simulink model "realisticversion"  (R2020b)
settings: Solver=VariableStepAuto  StartTime=0.0  StopTime=0.1  MaxStep=1e-7  RelTol=1e-3
undefined symbols (not defined in the file): Acid, Lead
libraries: fl_lib x63, powerlib x24, nesl_utility x22, ee_lib x14, electricdrivelib x1, powerlib_meascontrol x1
settings Model: SimulationMode=accelerator  Creator=ahmet  LastModifiedBy=90554
settings SolverCC: ZeroCrossAlgorithm=Adaptive
settings DataIOCC: ReturnWorkspaceOutputs=off
settings DebuggingCC: IgnoredZcDiagnostic=none

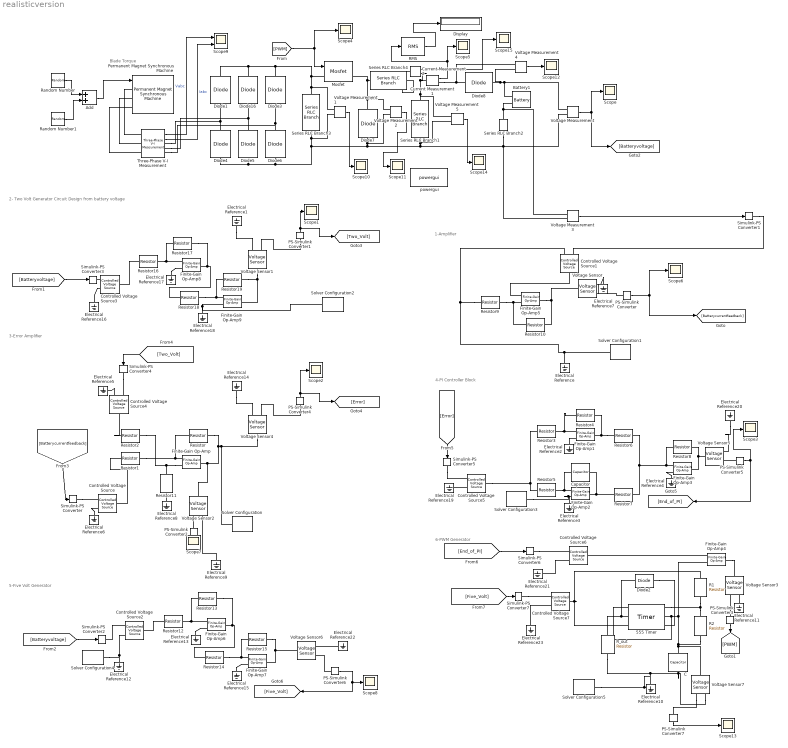
== system realisticversion ==
  note: 1-Amplifier
  note: 6-PWM Generator
  note: 5-Five Volt Generator
  note: 4-PI Controller Block
  note: 3-Error Amplifier
  note: 2- Two Volt Generator Circuit Design from battery voltage
  note: Blade Torque
  555 Timer : ee_lib/Integrated Circuits/Timer  V_CC=5 V  V_OL=0 V  V_OH=4.7 V  R_OUT=8 Ohm  Delay=1e-7 s  R_DIV=5 kOhm  R_closed=12 Ohm  R_open=5e+8 Ohm
      settings: SourceProductBaseCode=PS  InternalSimscapePortConfiguration="{\"Bottom\":[],\"Left\":[{\"id\":\"TRIG\",\"label\":\"TRIG\",\"type\":\"foundation.electrical.electrical\"},{\"id\":\"OUT\",\"label\":\"OUT\",\"type\":\"foundation.electrical.electrical\"},{\"id\":\"RESET\",\"label\":\"RESET\",\"type\":\"foundation.electrical.electrical\"}],\"Right\":[{\"id\":\"DISCH\",\"label\":\"DISCH\",\"type\":\"foundation.electrical.electrical\"},{\"id\":\"THRES\",\"label\":\"THRES\",\"type\":\"foundation.electrical.electrical\"},{\"id\":\"CONT\",\"label\":\"CONT\",\"type\":\"foundation.electrical.electrical\"}],\"Top\":[]}"
  Add : Sum
  Battery1 : electricdrivelib/Extra Sources/Battery  BatType=Lead-Acid  ShowTempParam=off  ThermalPreset=no  ShowAgeParam=off  NomV=24  NomQ=5.4  SOC=50  Batt_Tr=30  PresetModel=on  MaxQ=5.625  MinV=18  FullV=26.1316  Dis_rate=1.08  R=0.044444  Normal_OP=1.6755  expZone="[24.4342        0.018]"  current=[6.5 13 32.5]  Units=Time  Tci=20  NomT=20  T2=-30  MaxQ2=4.8  FullV2=7.1  Normal_OP2=5.655  expZone2="[6.58           1]"  Rca=0.6  ti=2000  Dp=0  Neq0=0  Tsim=1e6  Ta1=25  Qeol=5.4*0.9  Reol=0.013333*1.2  Char_age=[2.3478, 3]  Dis_age=[2.3478, 10]  N1=1500  N2=10500  N3=1000  N4=1400  Ta2=45  N5=950
  C : fl_lib/Electrical/Electrical Elements/Capacitor  c=1e-9 F  r=1e-6 Ohm  g=0 1/Ohm  i_specify=off  i_priority=None  i=0 A  i_nominal_specify=off  i_nominal_unit=A  i_nominal_value=1  v_specify=off  v_priority=None  v=0 V  v_nominal_specify=off  v_nominal_unit=V  v_nominal_value=1  vc_specify=off  vc_priority=High  vc=0 V  vc_nominal_specify=off  vc_nominal_unit=V  vc_nominal_value=1
  Capacitor : fl_lib/Electrical/Electrical Elements/Capacitor  c=3.3e-6 F  r=1e-6 Ohm  g=0 1/Ohm  i_specify=off  i_priority=None  i=0 A  i_nominal_specify=off  i_nominal_unit=A  i_nominal_value=1  v_specify=off  v_priority=None  v=0 V  v_nominal_specify=off  v_nominal_unit=V  v_nominal_value=1  vc_specify=off  vc_priority=High  vc=0 V  vc_nominal_specify=off  vc_nominal_unit=V  vc_nominal_value=1
  Controlled Voltage Source{,1..7} (8 alike) : fl_lib/Electrical/Electrical Sources/Controlled Voltage Source
  Current Measurement1 : powerlib/Measurements/Current Measurement  PhasorSimulation=off  OutputType=Complex  PSBequivalent=0
  Current Measurement2 : powerlib/Measurements/Current Measurement  PhasorSimulation=off  OutputType=Complex  PSBequivalent=0
  Diode{1,3..6,16} (6 alike) : powerlib/Power Electronics/Diode  Ron=0.001  Lon=0  Vf=1.1  IC=0  UseSnubber=0  Rs=1e5  Cs=inf  Measurements=off
  Diode2 : ee_lib/Semiconductors & Converters/Diode  ModelType=ee.enum.diode.modelType.pwl  IfMat=[.07, .12, .19, 1.75, 4.24, 7.32, 11.2; .16, .3, .72, 2.14, 4.02, 6.35, 9.12] A  TjVec=[25, 125] degC  VfVec=[.5, .7, .9, 1.3, 1.7, 2.1, 2.5] V  Vf=0.6 V  Ron=0.3 Ohm  Goff=1e-8 S  prmExp=1  I12=[ 0.0137 0.545 ] A  V12=[ 0.6 0.7 ] V  IS=1e-12 A  ec=1  I1=0.0137 A  V1=0.6 V  RS=0.01 Ohm  Tmeas=25 degC  N_series=1  N_parallel=1  Rz=0.3 Ohm  BV=inf V  C_param=1  CJ=5 pF  CJ0=5 pF  VJ=1 V  Mgrad=0.5  Vvec=[ 0.1 10 100 ] V  Cvec=[ 3.5 1 0.4 ] pF  FC=0.5  Q_param=ee.enum.diode.recoveryParam.off  iRM=-7.15 A  iF=4 A  didt=-750 A/us  trr_factor=3  trr=115 ns  Qrr=1500 s*uA  TT=50 ns  tau=100 ns  T_param=1  IS_T2=1.25e-7 A  I1_T2=0.245 A  V1_T2=0.5 V  Tmeas2=125 degC  EG_param=1  EG=1.11 eV  XTI_param=1  XTI=3  dBVdT=0 V/K  Tdevice=25 degC  i_specify=off  i_priority=None  i=0 A  i_nominal_specify=off  i_nominal_unit=A  i_nominal_value=1  v_specify=off  v_priority=None  v=0 V  v_nominal_specify=off  v_nominal_unit=V  v_nominal_value=1  i_capacitor_specify=off  i_capacitor_priority=None  i_capacitor=0 A  i_capacitor_nominal_specify=off  i_capacitor_nominal_unit=A  i_capacitor_nominal_value=1  v_capacitor_specify=off  v_capacitor_priority=None  v_capacitor=0 V  v_capacitor_nominal_specify=off  v_capacitor_nominal_unit=V  v_capacitor_nominal_value=1  power_dissipated_specify=off  power_dissipated_priority=None  power_dissipated=0 W  power_dissipated_nominal_specify=off  power_dissipated_nominal_unit=W  power_dissipated_nominal_value=1  thermal_network_parameterization=ee.enum.thermalNetworkTopology.cauer  Rth=[0, 10] K/W  Rth_Foster=[4, 6] K/W  thermal_mass_parameterization=ee.enum.thermalNetwork.timeconstant  thermal_mass=[0, 1] J/K  thermal_mass_Foster=[1.5, 3] J/K  thermal_time_constant=[0, 10] s  thermal_time_constant_Foster=[6, 18] s  thermal_mass_initial_temperatures=[25, 25] degC
  Diode7 : powerlib/Power Electronics/Diode  Ron=0.001  Lon=0  Vf=1.27  IC=0  UseSnubber=0  Rs=1e5  Cs=inf  Measurements=off
  Diode8 : powerlib/Power Electronics/Diode  Ron=0.001  Lon=0  Vf=0.63  IC=0  UseSnubber=0  Rs=1e5  Cs=inf  Measurements=off
  Display : Display
  Electrical Reference{,1..23} (24 alike) : fl_lib/Electrical/Electrical Elements/Electrical Reference
  Finite-Gain Op-Amp : ee_lib/Integrated Circuits/Finite-Gain Op-Amp  A=1000  Rin=1e6 Ohm  Rout=100 Ohm  Vmin=-15 V  Vmax=15 V  noise_mode=0  v_noise=30e-9 V/Hz^0.50000  noise_prm=1  i_noise=0.5e-12 A/Hz^0.50000  ip_noise=0.5e-12 A/Hz^0.50000  in_noise=0.5e-12 A/Hz^0.50000  sample_time=1e-3 s  repeatability=1  auto_seed_v=3516351732  auto_seed_ip=3127860819  auto_seed_in=755105624  user_seed_v=0  user_seed_ip=0  user_seed_in=0
      settings: SourceProductBaseCode=PS  InternalSimscapePortConfiguration="{\"Bottom\":[],\"Left\":[{\"id\":\"p\",\"label\":\"+\",\"type\":\"foundation.electrical.electrical\"},{\"id\":\"n\",\"label\":\"-\",\"type\":\"foundation.electrical.electrical\"}],\"Right\":[{\"id\":\"out\",\"label\":\"\",\"type\":\"foundation.electrical.electrical\"}],\"Top\":[]}"
  Finite-Gain Op-Amp1 : ee_lib/Integrated Circuits/Finite-Gain Op-Amp  A=1000  Rin=1e6 Ohm  Rout=100 Ohm  Vmin=-15 V  Vmax=15 V  noise_mode=0  v_noise=30e-9 V/Hz^0.50000  noise_prm=1  i_noise=0.5e-12 A/Hz^0.50000  ip_noise=0.5e-12 A/Hz^0.50000  in_noise=0.5e-12 A/Hz^0.50000  sample_time=1e-3 s  repeatability=1  auto_seed_v=1547781561  auto_seed_ip=810846759  auto_seed_in=5147076  user_seed_v=0  user_seed_ip=0  user_seed_in=0
      settings: SourceProductBaseCode=PS  InternalSimscapePortConfiguration="{\"Bottom\":[],\"Left\":[{\"id\":\"p\",\"label\":\"+\",\"type\":\"foundation.electrical.electrical\"},{\"id\":\"n\",\"label\":\"-\",\"type\":\"foundation.electrical.electrical\"}],\"Right\":[{\"id\":\"out\",\"label\":\"\",\"type\":\"foundation.electrical.electrical\"}],\"Top\":[]}"
  Finite-Gain Op-Amp2 : ee_lib/Integrated Circuits/Finite-Gain Op-Amp  A=1000  Rin=1e6 Ohm  Rout=100 Ohm  Vmin=-15 V  Vmax=15 V  noise_mode=0  v_noise=30e-9 V/Hz^0.50000  noise_prm=1  i_noise=0.5e-12 A/Hz^0.50000  ip_noise=0.5e-12 A/Hz^0.50000  in_noise=0.5e-12 A/Hz^0.50000  sample_time=1e-3 s  repeatability=1  auto_seed_v=1359011463  auto_seed_ip=3004832076  auto_seed_in=2685450550  user_seed_v=0  user_seed_ip=0  user_seed_in=0
      settings: SourceProductBaseCode=PS  InternalSimscapePortConfiguration="{\"Bottom\":[],\"Left\":[{\"id\":\"p\",\"label\":\"+\",\"type\":\"foundation.electrical.electrical\"},{\"id\":\"n\",\"label\":\"-\",\"type\":\"foundation.electrical.electrical\"}],\"Right\":[{\"id\":\"out\",\"label\":\"\",\"type\":\"foundation.electrical.electrical\"}],\"Top\":[]}"
  Finite-Gain Op-Amp3 : ee_lib/Integrated Circuits/Finite-Gain Op-Amp  A=1000  Rin=1e6 Ohm  Rout=100 Ohm  Vmin=-15 V  Vmax=15 V  noise_mode=0  v_noise=30e-9 V/Hz^0.50000  noise_prm=1  i_noise=0.5e-12 A/Hz^0.50000  ip_noise=0.5e-12 A/Hz^0.50000  in_noise=0.5e-12 A/Hz^0.50000  sample_time=1e-3 s  repeatability=1  auto_seed_v=2332434283  auto_seed_ip=1885650430  auto_seed_in=1234490714  user_seed_v=0  user_seed_ip=0  user_seed_in=0
      settings: SourceProductBaseCode=PS  InternalSimscapePortConfiguration="{\"Bottom\":[],\"Left\":[{\"id\":\"p\",\"label\":\"+\",\"type\":\"foundation.electrical.electrical\"},{\"id\":\"n\",\"label\":\"-\",\"type\":\"foundation.electrical.electrical\"}],\"Right\":[{\"id\":\"out\",\"label\":\"\",\"type\":\"foundation.electrical.electrical\"}],\"Top\":[]}"
  Finite-Gain Op-Amp4 : ee_lib/Integrated Circuits/Finite-Gain Op-Amp  A=1000  Rin=1e6 Ohm  Rout=100 Ohm  Vmin=-15 V  Vmax=15 V  noise_mode=0  v_noise=30e-9 V/Hz^0.50000  noise_prm=1  i_noise=0.5e-12 A/Hz^0.50000  ip_noise=0.5e-12 A/Hz^0.50000  in_noise=0.5e-12 A/Hz^0.50000  sample_time=1e-3 s  repeatability=1  auto_seed_v=3499211588  auto_seed_ip=3890346746  auto_seed_in=545404223  user_seed_v=0  user_seed_ip=0  user_seed_in=0
      settings: SourceProductBaseCode=PS  InternalSimscapePortConfiguration="{\"Bottom\":[],\"Left\":[{\"id\":\"p\",\"label\":\"+\",\"type\":\"foundation.electrical.electrical\"},{\"id\":\"n\",\"label\":\"-\",\"type\":\"foundation.electrical.electrical\"}],\"Right\":[{\"id\":\"out\",\"label\":\"\",\"type\":\"foundation.electrical.electrical\"}],\"Top\":[]}"
  Finite-Gain Op-Amp5 : ee_lib/Integrated Circuits/Finite-Gain Op-Amp  A=1000  Rin=1e6 Ohm  Rout=100 Ohm  Vmin=-15 V  Vmax=15 V  noise_mode=0  v_noise=30e-9 V/Hz^0.50000  noise_prm=1  i_noise=0.5e-12 A/Hz^0.50000  ip_noise=0.5e-12 A/Hz^0.50000  in_noise=0.5e-12 A/Hz^0.50000  sample_time=1e-3 s  repeatability=1  auto_seed_v=625085161  auto_seed_ip=584410010  auto_seed_in=3733581602  user_seed_v=0  user_seed_ip=0  user_seed_in=0
      settings: SourceProductBaseCode=PS  InternalSimscapePortConfiguration="{\"Bottom\":[],\"Left\":[{\"id\":\"p\",\"label\":\"+\",\"type\":\"foundation.electrical.electrical\"},{\"id\":\"n\",\"label\":\"-\",\"type\":\"foundation.electrical.electrical\"}],\"Right\":[{\"id\":\"out\",\"label\":\"\",\"type\":\"foundation.electrical.electrical\"}],\"Top\":[]}"
  Finite-Gain Op-Amp6 : ee_lib/Integrated Circuits/Finite-Gain Op-Amp  A=1000  Rin=1e6 Ohm  Rout=100 Ohm  Vmin=-15 V  Vmax=15 V  noise_mode=0  v_noise=30e-9 V/Hz^0.50000  noise_prm=1  i_noise=0.5e-12 A/Hz^0.50000  ip_noise=0.5e-12 A/Hz^0.50000  in_noise=0.5e-12 A/Hz^0.50000  sample_time=1e-3 s  repeatability=1  auto_seed_v=591687118  auto_seed_ip=3593696983  auto_seed_in=595289837  user_seed_v=0  user_seed_ip=0  user_seed_in=0
      settings: SourceProductBaseCode=PS  InternalSimscapePortConfiguration="{\"Bottom\":[],\"Left\":[{\"id\":\"p\",\"label\":\"+\",\"type\":\"foundation.electrical.electrical\"},{\"id\":\"n\",\"label\":\"-\",\"type\":\"foundation.electrical.electrical\"}],\"Right\":[{\"id\":\"out\",\"label\":\"\",\"type\":\"foundation.electrical.electrical\"}],\"Top\":[]}"
  Finite-Gain Op-Amp7 : ee_lib/Integrated Circuits/Finite-Gain Op-Amp  A=1000  Rin=1e6 Ohm  Rout=100 Ohm  Vmin=-15 V  Vmax=15 V  noise_mode=0  v_noise=30e-9 V/Hz^0.50000  noise_prm=1  i_noise=0.5e-12 A/Hz^0.50000  ip_noise=0.5e-12 A/Hz^0.50000  in_noise=0.5e-12 A/Hz^0.50000  sample_time=1e-3 s  repeatability=1  auto_seed_v=2526340073  auto_seed_ip=1572631483  auto_seed_in=3465005860  user_seed_v=0  user_seed_ip=0  user_seed_in=0
      settings: SourceProductBaseCode=PS  InternalSimscapePortConfiguration="{\"Bottom\":[],\"Left\":[{\"id\":\"p\",\"label\":\"+\",\"type\":\"foundation.electrical.electrical\"},{\"id\":\"n\",\"label\":\"-\",\"type\":\"foundation.electrical.electrical\"}],\"Right\":[{\"id\":\"out\",\"label\":\"\",\"type\":\"foundation.electrical.electrical\"}],\"Top\":[]}"
  Finite-Gain Op-Amp8 : ee_lib/Integrated Circuits/Finite-Gain Op-Amp  A=1000  Rin=1e6 Ohm  Rout=100 Ohm  Vmin=-15 V  Vmax=15 V  noise_mode=0  v_noise=30e-9 V/Hz^0.50000  noise_prm=1  i_noise=0.5e-12 A/Hz^0.50000  ip_noise=0.5e-12 A/Hz^0.50000  in_noise=0.5e-12 A/Hz^0.50000  sample_time=1e-3 s  repeatability=1  auto_seed_v=3610853119  auto_seed_ip=1092133643  auto_seed_in=3497326697  user_seed_v=0  user_seed_ip=0  user_seed_in=0
      settings: SourceProductBaseCode=PS  InternalSimscapePortConfiguration="{\"Bottom\":[],\"Left\":[{\"id\":\"p\",\"label\":\"+\",\"type\":\"foundation.electrical.electrical\"},{\"id\":\"n\",\"label\":\"-\",\"type\":\"foundation.electrical.electrical\"}],\"Right\":[{\"id\":\"out\",\"label\":\"\",\"type\":\"foundation.electrical.electrical\"}],\"Top\":[]}"
  Finite-Gain Op-Amp9 : ee_lib/Integrated Circuits/Finite-Gain Op-Amp  A=1000  Rin=1e6 Ohm  Rout=100 Ohm  Vmin=-15 V  Vmax=15 V  noise_mode=0  v_noise=30e-9 V/Hz^0.50000  noise_prm=1  i_noise=0.5e-12 A/Hz^0.50000  ip_noise=0.5e-12 A/Hz^0.50000  in_noise=0.5e-12 A/Hz^0.50000  sample_time=1e-3 s  repeatability=1  auto_seed_v=1045931777  auto_seed_ip=3991156871  auto_seed_in=1503168829  user_seed_v=0  user_seed_ip=0  user_seed_in=0
      settings: SourceProductBaseCode=PS  InternalSimscapePortConfiguration="{\"Bottom\":[],\"Left\":[{\"id\":\"p\",\"label\":\"+\",\"type\":\"foundation.electrical.electrical\"},{\"id\":\"n\",\"label\":\"-\",\"type\":\"foundation.electrical.electrical\"}],\"Right\":[{\"id\":\"out\",\"label\":\"\",\"type\":\"foundation.electrical.electrical\"}],\"Top\":[]}"
  Mosfet : powerlib/Power Electronics/Mosfet  Ron=0.1  Lon=0  Rd=0.01  Vfd=0  IC=0  Rs=1e5  Cs=inf  Measurements=on
  PS-Simulink Converter : nesl_utility/PS-Simulink Converter  PhysicalDomain=network_engine_domain  SubClassName=ps_output  LeftPortType=input  RightPortType=output  PseudoPeriodic=off  Frequencies=[]  Unit=1  AffineConversion=off
  PS-Simulink Converter{1..7} (7 alike) : nesl_utility/PS-Simulink Converter  PhysicalDomain=network_engine_domain  SubClassName=ps_output  LeftPortType=input  RightPortType=output  PseudoPeriodic=off  Frequencies=[]  Unit=inherit  AffineConversion=off
  Permanent Magnet Synchronous Machine : powerlib/Machines/Permanent Magnet Synchronous Machine  NbPhases=3  FluxDistribution=Sinusoidal  RotorType=Round  MechanicalLoad=Torque Tm  PresetModel=No  ShowDetailedParameters=on  MeasurementBus=off  Resistance=10.58  Inductance=8.5e-3  dqInductances=[8.5e-3,8.5e-3]  La=0.0167  MachineConstant=Voltage Constant (V_peak L-L / krpm)  Flux=0.60646  VoltageCst=110  TorqueCst=0.90969  Flat=120  Mechanical=[0.00027 0.005024 1 0]  PolePairs=4  InitialConditions=[300,0, 0,0]  InitialConditions5ph=[0 0 0 0 0 0]  RefAngle=90 degrees behind phase A axis (modified Park)  IterativeDiscreteModel=Trapezoidal non iterative  TsBlock=-1  TsPowergui=0
  R1 : fl_lib/Electrical/Electrical Elements/Resistor  R=100e3 Ohm  i_specify=off  i_priority=None  i=0 A  i_nominal_specify=off  i_nominal_unit=A  i_nominal_value=1  v_specify=off  v_priority=None  v=0 V  v_nominal_specify=off  v_nominal_unit=V  v_nominal_value=1
  R2 : fl_lib/Electrical/Electrical Elements/Resistor  R=3.3e3 Ohm  i_specify=off  i_priority=None  i=0 A  i_nominal_specify=off  i_nominal_unit=A  i_nominal_value=1  v_specify=off  v_priority=None  v=0 V  v_nominal_specify=off  v_nominal_unit=V  v_nominal_value=1
  RMS : powerlib_meascontrol/Measurements/RMS  TrueRMS=on  Freq=60  RMSInit=120  Ts=0
  R_out : fl_lib/Electrical/Electrical Elements/Resistor  R=1.2e3 Ohm  i_specify=off  i_priority=None  i=0 A  i_nominal_specify=off  i_nominal_unit=A  i_nominal_value=1  v_specify=off  v_priority=None  v=0 V  v_nominal_specify=off  v_nominal_unit=V  v_nominal_value=1
  Random Number : RandomNumber  Mean=-1.6  Variance=0.05  SampleTime=1
  Random Number1 : RandomNumber  Variance=0.1  SampleTime=1e-3
  Resistor{,1,14..15,18..19} (6 alike) : fl_lib/Electrical/Electrical Elements/Resistor  R=5.1e3 Ohm  i_specify=off  i_priority=None  i=0 A  i_nominal_specify=off  i_nominal_unit=A  i_nominal_value=1  v_specify=off  v_priority=None  v=0 V  v_nominal_specify=off  v_nominal_unit=V  v_nominal_value=1
  Resistor10 : ee_lib/Passive/Resistor  R=1.2e3 Ohm  R_tol=5  enable_R_tol=0  tol_distribution=1  nSigma=4  enable_operating_limits=0  operating_limit_action=2  max_working_voltage=100 V  power_rating=1 W  enable_faults=0  fault_action=1  R_faulted=inf Ohm  enable_temporal_fault=0  t_fault=1 s  enable_behavioral_fault=0  max_permissible_current=1 A  t_fail_on_current=1 s  noise_mode=0  sample_time=1e-3 s  repeatability=1  auto_seed=3499211588  user_seed=0  Tdevice=25 degC  alpha=3.93e-3 1/K  Tmeas=25 degC  thermal_mass=100 J/K  power_derating_T1=70 degC  power_derating_T2=155 degC  operating_temperature_range_vec=[-50, 150] degC  temperature_specify=off  temperature_priority=High  temperature=298.15 K  temperature_nominal_specify=off  temperature_nominal_unit=K  temperature_nominal_value=1
  Resistor11 : fl_lib/Electrical/Electrical Elements/Resistor  R=3.3e3 Ohm  i_specify=off  i_priority=None  i=0 A  i_nominal_specify=off  i_nominal_unit=A  i_nominal_value=1  v_specify=off  v_priority=None  v=0 V  v_nominal_specify=off  v_nominal_unit=V  v_nominal_value=1
  Resistor12 : fl_lib/Electrical/Electrical Elements/Resistor  R=2.7e3 Ohm  i_specify=off  i_priority=None  i=0 A  i_nominal_specify=off  i_nominal_unit=A  i_nominal_value=1  v_specify=off  v_priority=None  v=0 V  v_nominal_specify=off  v_nominal_unit=V  v_nominal_value=1
  Resistor13 : fl_lib/Electrical/Electrical Elements/Resistor  R=560 Ohm  i_specify=off  i_priority=None  i=0 A  i_nominal_specify=off  i_nominal_unit=A  i_nominal_value=1  v_specify=off  v_priority=None  v=0 V  v_nominal_specify=off  v_nominal_unit=V  v_nominal_value=1
  Resistor16 : fl_lib/Electrical/Electrical Elements/Resistor  R=12e3 Ohm  i_specify=off  i_priority=None  i=0 A  i_nominal_specify=off  i_nominal_unit=A  i_nominal_value=1  v_specify=off  v_priority=None  v=0 V  v_nominal_specify=off  v_nominal_unit=V  v_nominal_value=1
  Resistor17 : fl_lib/Electrical/Electrical Elements/Resistor  R=1e3 Ohm  i_specify=off  i_priority=None  i=0 A  i_nominal_specify=off  i_nominal_unit=A  i_nominal_value=1  v_specify=off  v_priority=None  v=0 V  v_nominal_specify=off  v_nominal_unit=V  v_nominal_value=1
  Resistor2 : fl_lib/Electrical/Electrical Elements/Resistor  R=1.2e3 Ohm  i_specify=off  i_priority=None  i=0 A  i_nominal_specify=off  i_nominal_unit=A  i_nominal_value=1  v_specify=off  v_priority=None  v=0 V  v_nominal_specify=off  v_nominal_unit=V  v_nominal_value=1
  Resistor3 : fl_lib/Electrical/Electrical Elements/Resistor  R=5.6e3 Ohm  i_specify=off  i_priority=None  i=0 A  i_nominal_specify=off  i_nominal_unit=A  i_nominal_value=1  v_specify=off  v_priority=None  v=0 V  v_nominal_specify=off  v_nominal_unit=V  v_nominal_value=1
  Resistor4 : fl_lib/Electrical/Electrical Elements/Resistor  R=680 Ohm  i_specify=off  i_priority=None  i=0 A  i_nominal_specify=off  i_nominal_unit=A  i_nominal_value=1  v_specify=off  v_priority=None  v=0 V  v_nominal_specify=off  v_nominal_unit=V  v_nominal_value=1
  Resistor5 : fl_lib/Electrical/Electrical Elements/Resistor  R=2.2e3 Ohm  i_specify=off  i_priority=None  i=0 A  i_nominal_specify=off  i_nominal_unit=A  i_nominal_value=1  v_specify=off  v_priority=None  v=0 V  v_nominal_specify=off  v_nominal_unit=V  v_nominal_value=1
  Resistor6 : fl_lib/Electrical/Electrical Elements/Resistor  R=820 Ohm  i_specify=off  i_priority=None  i=0 A  i_nominal_specify=off  i_nominal_unit=A  i_nominal_value=1  v_specify=off  v_priority=None  v=0 V  v_nominal_specify=off  v_nominal_unit=V  v_nominal_value=1
  Resistor7 : fl_lib/Electrical/Electrical Elements/Resistor  R=820 Ohm  i_specify=off  i_priority=None  i=0 A  i_nominal_specify=off  i_nominal_unit=A  i_nominal_value=1  v_specify=off  v_priority=None  v=0 V  v_nominal_specify=off  v_nominal_unit=V  v_nominal_value=1
  Resistor8 : fl_lib/Electrical/Electrical Elements/Resistor  R=2.2e3 Ohm  i_specify=off  i_priority=None  i=0 A  i_nominal_specify=off  i_nominal_unit=A  i_nominal_value=1  v_specify=off  v_priority=None  v=0 V  v_nominal_specify=off  v_nominal_unit=V  v_nominal_value=1
  Resistor9 : ee_lib/Passive/Resistor  R=240 Ohm  R_tol=5  enable_R_tol=0  tol_distribution=1  nSigma=4  enable_operating_limits=0  operating_limit_action=2  max_working_voltage=100 V  power_rating=1 W  enable_faults=0  fault_action=1  R_faulted=inf Ohm  enable_temporal_fault=0  t_fault=1 s  enable_behavioral_fault=0  max_permissible_current=1 A  t_fail_on_current=1 s  noise_mode=0  sample_time=1e-3 s  repeatability=1  auto_seed=3890346746  user_seed=0  Tdevice=25 degC  alpha=3.93e-3 1/K  Tmeas=25 degC  thermal_mass=100 J/K  power_derating_T1=70 degC  power_derating_T2=155 degC  operating_temperature_range_vec=[-50, 150] degC  temperature_specify=off  temperature_priority=High  temperature=298.15 K  temperature_nominal_specify=off  temperature_nominal_unit=K  temperature_nominal_value=1
      settings: SourceProductBaseCode=SN
  Scope{,1..8,10..15} (15 alike) : Scope
  Scope9 : Scope  NumInputPorts=2
  Series RLC Branch1 : powerlib/Elements/Series RLC Branch  LConnTagsString=__new0  RConnTagsString=__new0  BranchType=C  Resistance=1  Inductance=5.5e-3  SetiL0=off  InitialCurrent=0  Capacitance=100e-6  Setx0=off  InitialVoltage=24  Measurements=None
  Series RLC Branch2 : powerlib/Elements/Series RLC Branch  LConnTagsString=__new0  RConnTagsString=__new0  BranchType=R  Resistance=0.25  Inductance=5.5e-3  SetiL0=off  InitialCurrent=0  Capacitance=2e-3  Setx0=off  InitialVoltage=0  Measurements=None
  Series RLC Branch3 : powerlib/Elements/Series RLC Branch  LConnTagsString=__new0  RConnTagsString=__new0  BranchType=C  Resistance=1  Inductance=5.5e-3  SetiL0=off  InitialCurrent=0  Capacitance=1e-4  Setx0=off  InitialVoltage=0  Measurements=None
  Series RLC Branch4 : powerlib/Elements/Series RLC Branch  LConnTagsString=__new0  RConnTagsString=__new0  BranchType=L  Resistance=1  Inductance=15e-3  SetiL0=off  InitialCurrent=2  Capacitance=1e-6  Setx0=off  InitialVoltage=0  Measurements=None
  Simulink-PS Converter{,1..7} (8 alike) : nesl_utility/Simulink-PS Converter  PhysicalDomain=network_engine_domain  SubClassName=ps_input  LeftPortType=input  RightPortType=output  PseudoPeriodic=off  Frequencies=[]  NoiseDistribution=none  NoiseParameters=[]  Unit=1  AffineConversion=off  FilteringAndDerivatives=provide  SimscapeFilterOrder=1  InputFilterTimeConstant=0.001  UdotUserProvided=0
  Solver Configuration{,1..5} (6 alike) : nesl_utility/Solver Configuration  PhysicalDomain=network_engine_domain  SubClassName=solver  LeftPortType=input  RightPortType=generic  Tones=[]  Harmonics=[]  SimulateNoise=off  Profile=off  UseLocalSampling=off  EnableSwitchedLinearOptims=on  FrequencyDomain=off  UseCCode=off  RelTol=0.001  AbsTol=1e-06  MinStep=1e-09  ToWorkspace=off  RevertToSquareIcSolve=off  NumHomotopyIterations=100  PhasorMode=off  PhasorModeNumHarmonics=1  DoDC=off  ResidualTolerance=1e-09  UseLocalSolver=off  LocalSolverChoice=NE_BACKWARD_EULER_ADVANCER  LocalSolverSampleTime=0.001  DoFixedCost=off  MaxNonlinIter=3  MaxModeIter=2  ComputeImpulses=off  ImpulseIterations=2  LinearAlgebra=auto  EquationFormulation=NE_TIME_EF  DelaysMemoryBudget=1024  AutomaticFiltering=on  FilteringTimeConstant=0.001  PartitionStorageMethod=AS_NEEDED  PartitionMemoryBudget=1024  PartitionMethod=ROBUST
  Three-Phase V-I Measurement : powerlib/Measurements/Three-Phase V-I Measurement  VoltageMeasurement=phase-to-phase  SetLabelV=off  LabelV=Vabc  Vpu=off  VpuLL=off  CurrentMeasurement=yes  SetLabelI=off  LabelI=Iabc  Ipu=off  Pbase=100e6  Vbase=500e3  OutputType=Complex  PhasorSimulation=off  PSBequivalent=0
  Voltage Measurement{,1..5} (6 alike) : powerlib/Measurements/Voltage Measurement  PhasorSimulation=off  OutputType=Complex  PSBequivalent=0
  Voltage Sensor{,1..7} (8 alike) : fl_lib/Electrical/Electrical Sensors/Voltage Sensor
  powergui : powerlib/powergui  Priority=1  SimulationMode=Continuous  SampleTime=1e-7  frequency=60  Iterations=50  frequencyindice=0  Pbase=100e6  ErrMax=1e-4  UnitsV=kV  UnitsW=MW  buscounter=0  FunctionMessages=off  echomessages=off  EnableUseOfTLC=off  CurrentSourceSwitches=off  DisableSnubberDevices=off  DisableRonSwitches=off  DisableVfSwitches=off  DisplayEquations=off  AutomaticDiscreteSolvers=off  SolverType=Tustin/Backward Euler (TBE)  Interpol=off  ExternalGateDelay=off  methode=off  Ts=100  x0status=blocks  SPID=on  SwTol=0  HookPort=off  NonlinearTolerance=1e-4  nMaxIteration=100  ContinueOnMaxIteration=off  RestoreLinks=warning  ResistiveCurrentMeasurement=off  Frange=[0:2:500]  Ylog=off  Xlog=on  ShowGrid=off  save=off  variable=ZData  structure=ScopeData  ZoomFFT=off  StartTime=0.1  cycles=100  DisplayStyle=1  fundamental=10000  FreqAxis=off  MaxFrequency=10000  frequencyindicesteady=1  RmsSteady=1  display=off
  wires:
  [PWM] -> Scope4/1, Mosfet/1
  Voltage Measurement/1 -> Scope/1, [Batteryvoltage]
  Random Number/1 -> Add/1
  Add/1 -> Permanent Magnet Synchronous Machine/1
  Random Number1/1 -> Add/2
  PS-Simulink Converter3/1 -> [PWM]
  Voltage Measurement3/1 -> Simulink-PS Converter1/1
  PS-Simulink Converter/1 -> [Batterycurrentfeedback], Scope6/1
  Current Measurement1/1 -> RMS/1, Scope5/1
  RMS/1 -> Display/1
  [Batterycurrentfeedback] -> Simulink-PS Converter/1
  PS-Simulink Converter2/1 -> Scope7/1
  [Batteryvoltage] -> Simulink-PS Converter2/1
  [Batteryvoltage] -> Simulink-PS Converter3/1
  PS-Simulink Converter1/1 -> [Two_Volt], Scope1/1
  [Two_Volt] -> Simulink-PS Converter4/1
  PS-Simulink Converter4/1 -> Scope2/1, [Error]
  [Error] -> Simulink-PS Converter5/1
  PS-Simulink Converter5/1 -> Scope3/1, [End_of_PI]
  [End_of_PI] -> Simulink-PS Converter6/1
  PS-Simulink Converter6/1 -> [Five_Volt], Scope8/1
  [Five_Volt] -> Simulink-PS Converter7/1
  Three-Phase V-I Measurement/1 -> Scope9/1  "Vabc"
  Three-Phase V-I Measurement/2 -> Scope9/2  "Iabc"
  Voltage Measurement1/1 -> Scope10/1
  Voltage Measurement2/1 -> Scope11/1
  Voltage Measurement4/1 -> Scope12/1
  PS-Simulink Converter7/1 -> Scope13/1
  Voltage Measurement5/1 -> Scope14/1
  Current Measurement2/1 -> Scope15/1
  connections:
  Diode1/RConn1 -- Voltage Measurement1/LConn1 -- Series RLC Branch3/LConn1 -- Mosfet/LConn1 -- Diode3/RConn1 -- Diode16/RConn1
  Voltage Measurement5/LConn1 -- Series RLC Branch1/LConn1 -- Current Measurement2/RConn1 -- Current Measurement1/LConn1
  Diode7/RConn1 -- Series RLC Branch4/LConn1 -- Mosfet/RConn1 -- Voltage Measurement2/LConn1
  Current Measurement1/RConn1 -- Voltage Measurement4/LConn1 -- Diode8/LConn1
  Diode8/RConn1 -- Voltage Measurement4/LConn2 -- Battery1/LConn1 -- Voltage Measurement/LConn1
  R2/RConn1 -- 555 Timer/RConn2 -- 555 Timer/LConn1 -- Finite-Gain Op-Amp4/LConn2 -- Voltage Sensor7/LConn1 -- C/LConn1
  R_out/RConn1 -- Voltage Sensor7/RConn2 -- C/RConn1 -- Electrical Reference10/LConn1 -- Solver Configuration5/RConn1
  555 Timer/LConn2 -- R_out/LConn1 -- Diode2/RConn1
  R2/LConn1 -- R1/RConn1 -- 555 Timer/RConn1
  Diode2/LConn1 -- 555 Timer/RConn3
  Electrical Reference11/LConn1 -- Voltage Sensor3/RConn2
  PS-Simulink Converter3/LConn1 -- Voltage Sensor3/RConn1
  Finite-Gain Op-Amp4/RConn1 -- Voltage Sensor3/LConn1
  Battery1/LConn2 -- Voltage Measurement3/LConn1 -- Series RLC Branch2/LConn1
  Resistor10/LConn1 -- Finite-Gain Op-Amp5/LConn2 -- Resistor9/RConn1
  Voltage Sensor/LConn1 -- Resistor10/RConn1 -- Finite-Gain Op-Amp5/RConn1
  Resistor9/LConn1 -- Solver Configuration1/RConn1 -- Electrical Reference/LConn1 -- Controlled Voltage Source1/RConn2
  PS-Simulink Converter/LConn1 -- Voltage Sensor/RConn1
  Finite-Gain Op-Amp5/LConn1 -- Controlled Voltage Source1/LConn1
  Simulink-PS Converter1/RConn1 -- Controlled Voltage Source1/RConn1
  Electrical Reference7/LConn1 -- Voltage Sensor/RConn2
  Diode4/LConn1 -- Voltage Measurement5/LConn2 -- Series RLC Branch1/RConn1 -- Series RLC Branch2/RConn1 -- Voltage Measurement/LConn2 -- Voltage Measurement3/LConn2 -- Voltage Measurement2/LConn2 -- Diode7/LConn1 -- Voltage Measurement1/LConn2 -- Series RLC Branch3/RConn1 -- Diode6/LConn1 -- Diode5/LConn1
  Diode6/RConn1 -- Diode3/LConn1 -- Three-Phase V-I Measurement/RConn3
  Diode5/RConn1 -- Diode16/LConn1 -- Three-Phase V-I Measurement/RConn2
  Diode4/RConn1 -- Diode1/LConn1 -- Three-Phase V-I Measurement/RConn1
  Controlled Voltage Source2/RConn1 -- Simulink-PS Converter2/RConn1
  Electrical Reference12/LConn1 -- Solver Configuration4/RConn1 -- Controlled Voltage Source2/RConn2
  Resistor12/RConn1 -- Finite-Gain Op-Amp6/LConn1 -- Resistor13/LConn1
  Finite-Gain Op-Amp6/LConn2 -- Electrical Reference13/LConn1
  Resistor12/LConn1 -- Controlled Voltage Source2/LConn1
  R1/LConn1 -- Controlled Voltage Source7/LConn1 -- 555 Timer/LConn3
  Finite-Gain Op-Amp7/LConn1 -- Resistor14/RConn1 -- Resistor15/LConn1
  Finite-Gain Op-Amp7/LConn2 -- Electrical Reference15/LConn1
  Resistor14/LConn1 -- Resistor13/RConn1 -- Finite-Gain Op-Amp6/RConn1
  Finite-Gain Op-Amp/LConn2 -- Resistor1/RConn1 -- Resistor/LConn1
  Resistor3/LConn1 -- Controlled Voltage Source5/LConn1 -- Resistor5/LConn1
  Finite-Gain Op-Amp1/LConn2 -- Resistor4/LConn1 -- Resistor3/RConn1
  Finite-Gain Op-Amp/LConn1 -- Resistor2/RConn1 -- Resistor11/LConn1
  Resistor8/RConn1 -- Voltage Sensor5/LConn1 -- Finite-Gain Op-Amp3/RConn1
  Resistor7/RConn1 -- Resistor6/RConn1 -- Resistor8/LConn1 -- Finite-Gain Op-Amp3/LConn2
  Resistor6/LConn1 -- Resistor4/RConn1 -- Finite-Gain Op-Amp1/RConn1
  Resistor7/LConn1 -- Capacitor/RConn1 -- Finite-Gain Op-Amp2/RConn1
  Capacitor/LConn1 -- Resistor5/RConn1 -- Finite-Gain Op-Amp2/LConn2
  Controlled Voltage Source/RConn2 -- Electrical Reference6/LConn1
  Finite-Gain Op-Amp3/LConn1 -- Electrical Reference4/LConn1
  Simulink-PS Converter/RConn1 -- Controlled Voltage Source/RConn1
  Finite-Gain Op-Amp2/LConn1 -- Solver Configuration3/RConn1 -- Electrical Reference3/LConn1
  Electrical Reference9/LConn1 -- Voltage Sensor2/RConn2
  PS-Simulink Converter2/LConn1 -- Voltage Sensor2/RConn1
  Electrical Reference8/LConn1 -- Resistor11/RConn1
  Resistor1/LConn1 -- Controlled Voltage Source/LConn1
  Finite-Gain Op-Amp1/LConn1 -- Electrical Reference2/LConn1
  Resistor16/RConn1 -- Resistor17/LConn1 -- Finite-Gain Op-Amp8/LConn1
  Finite-Gain Op-Amp9/LConn1 -- Resistor19/LConn1 -- Resistor18/RConn1
  Resistor18/LConn1 -- Finite-Gain Op-Amp8/RConn1 -- Resistor17/RConn1
  Finite-Gain Op-Amp8/LConn2 -- Electrical Reference17/LConn1
  Electrical Reference16/LConn1 -- Controlled Voltage Source3/RConn2
  Resistor16/LConn1 -- Controlled Voltage Source3/LConn1
  Finite-Gain Op-Amp9/LConn2 -- Solver Configuration2/RConn1 -- Electrical Reference18/LConn1
  Controlled Voltage Source3/RConn1 -- Simulink-PS Converter3/RConn1
  Resistor19/RConn1 -- Voltage Sensor1/LConn1 -- Finite-Gain Op-Amp9/RConn1
  PS-Simulink Converter1/LConn1 -- Voltage Sensor1/RConn1
  Electrical Reference1/LConn1 -- Voltage Sensor1/RConn2
  Simulink-PS Converter4/RConn1 -- Controlled Voltage Source4/RConn1
  Controlled Voltage Source4/RConn2 -- Electrical Reference5/LConn1
  Resistor2/LConn1 -- Controlled Voltage Source4/LConn1
  Voltage Sensor2/LConn1 -- Voltage Sensor4/LConn1 -- Solver Configuration/RConn1 -- Resistor/RConn1 -- Finite-Gain Op-Amp/RConn1
  PS-Simulink Converter4/LConn1 -- Voltage Sensor4/RConn1
  Electrical Reference14/LConn1 -- Voltage Sensor4/RConn2
  Simulink-PS Converter5/RConn1 -- Controlled Voltage Source5/RConn1
  Controlled Voltage Source5/RConn2 -- Electrical Reference19/LConn1
  Electrical Reference20/LConn1 -- Voltage Sensor5/RConn2
  PS-Simulink Converter5/LConn1 -- Voltage Sensor5/RConn1
  Controlled Voltage Source6/RConn2 -- Electrical Reference21/LConn1
  Simulink-PS Converter6/RConn1 -- Controlled Voltage Source6/RConn1
  Finite-Gain Op-Amp4/LConn1 -- Controlled Voltage Source6/LConn1
  Resistor15/RConn1 -- Finite-Gain Op-Amp7/RConn1 -- Voltage Sensor6/LConn1
  Electrical Reference22/LConn1 -- Voltage Sensor6/RConn2
  PS-Simulink Converter6/LConn1 -- Voltage Sensor6/RConn1
  Controlled Voltage Source7/RConn2 -- Electrical Reference23/LConn1
  Simulink-PS Converter7/RConn1 -- Controlled Voltage Source7/RConn1
  Permanent Magnet Synchronous Machine/LConn1 -- Three-Phase V-I Measurement/LConn1
  Permanent Magnet Synchronous Machine/LConn2 -- Three-Phase V-I Measurement/LConn2
  Permanent Magnet Synchronous Machine/LConn3 -- Three-Phase V-I Measurement/LConn3
  Voltage Sensor7/RConn1 -- PS-Simulink Converter7/LConn1
  Current Measurement2/LConn1 -- Series RLC Branch4/RConn1
